simulink model "LIN_1DOF"  (R2019b)
settings: Solver=VariableStepAuto  StartTime=0.0  StopTime=600  RelTol=1e-3
InitFcn:
  | load("parameters.mat")
  | load("Coefficients.mat")
undefined symbols (not defined in the file): Dm, Dt, g, Jeq, Jp, k_pitch_, Mb, w_ramp_0N, w_ramp_0P, w_ramp_1N, w_ramp_1P
libraries: cstblocks x2
settings Model: Creator=laptop  LastModifiedBy=lbend
settings OptimizationCC: BlockReduction=off  DefaultParameterBehavior=Inlined  BufferReuse=off

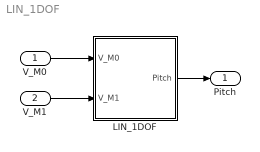
== system LIN_1DOF ==
  "V_M0 " : Inport
  V_M1 : Inport  Port=2
  LIN_1DOF : Subsystem
  Pitch : Outport
  wires:
  "V_M0 "/1 -> LIN_1DOF/1("V_M0 ")
  V_M1/1 -> LIN_1DOF/2(V_M1)
  LIN_1DOF/1(Pitch) -> Pitch/1

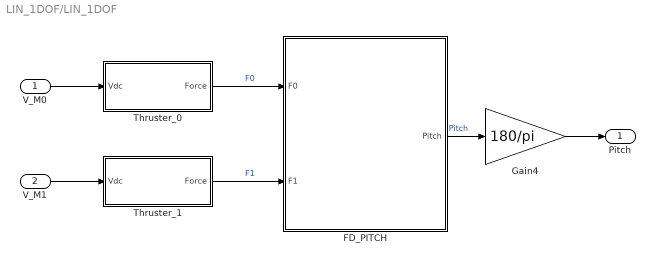
== system LIN_1DOF/LIN_1DOF ==
  "V_M0 " : Inport
  V_M1 : Inport  Port=2
  FD_PITCH : Subsystem
  Gain4 : Gain  Gain=180/pi
  Thruster_0 : Subsystem
  "Thruster_1 " : Subsystem
  Pitch : Outport
  wires:
  Thruster_0/1(Force) -> FD_PITCH/1(F0)  "F0"
  "Thruster_1 "/1(Force) -> FD_PITCH/2(F1)  "F1"
  V_M1/1 -> "Thruster_1 "/1(Vdc)
  "V_M0 "/1 -> Thruster_0/1(Vdc)
  FD_PITCH/1(Pitch) -> Gain4/1  "Pitch"
  Gain4/1 -> Pitch/1

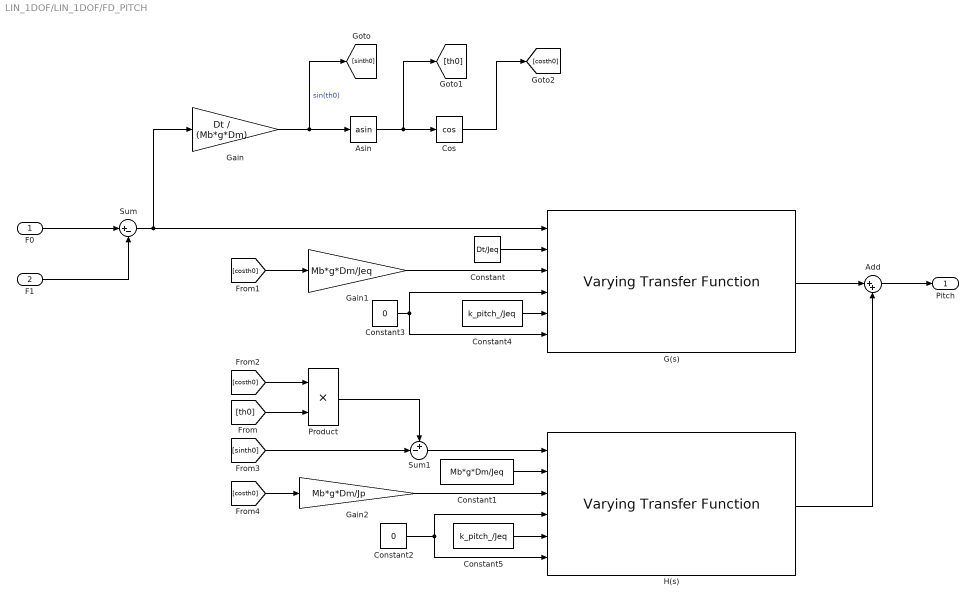
== system LIN_1DOF/LIN_1DOF/FD_PITCH ==
  F0 : Inport
  F1 : Inport  Port=2
  Add : Sum  Inputs=|++
  Asin : Trigonometry  Operator=asin
  Constant : Constant  Value=Dt/Jeq
  Constant1 : Constant  Value=Mb*g*Dm/Jeq
  Constant2 : Constant  Value=0
  Constant3 : Constant  Value=0
  Constant4 : Constant  Value=k_pitch_/Jeq
  Constant5 : Constant  Value=k_pitch_/Jeq
  Cos : Trigonometry  Operator=cos
  G(s) : cstblocks/Linear Parameter Varying/Varying Transfer Function  N=2
      settings: SourceProductName=Control System Toolbox
  Gain : Gain  Gain=Dt / (Mb*g*Dm)
  Gain1 : Gain  Gain=Mb*g*Dm/Jeq
  Gain2 : Gain  Gain=Mb*g*Dm/Jp
  H(s) : cstblocks/Linear Parameter Varying/Varying Transfer Function  N=2
      settings: SourceProductName=Control System Toolbox
  Product : Product
  Sum : Sum  Inputs=|+-
  Sum1 : Sum  Inputs=+-|
  Pitch : Outport
  wires:
  F1/1 -> Sum/2
  Constant1/1 -> H(s)/2
  Gain/1 -> [sinth0], Asin/1  "sin(th0)"
  Constant2/1 -> H(s)/6, H(s)/4
  Asin/1 -> [th0], Cos/1
  Gain2/1 -> H(s)/3
  [sinth0] -> Sum1/2
  Sum/1 -> G(s)/1, Gain/1
  Constant4/1 -> G(s)/5
  Product/1 -> Sum1/1
  [costh0] -> Gain1/1
  [th0] -> Product/2
  H(s)/1 -> Add/2
  F0/1 -> Sum/1
  [costh0] -> Product/1
  Constant/1 -> G(s)/2
  Constant3/1 -> G(s)/6, G(s)/4
  Gain1/1 -> G(s)/3
  [costh0] -> Gain2/1
  Constant5/1 -> H(s)/5
  Cos/1 -> [costh0]
  G(s)/1 -> Add/1
  Sum1/1 -> H(s)/1
  Add/1 -> Pitch/1

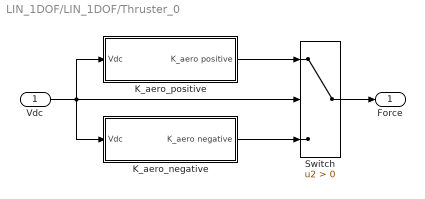
== system LIN_1DOF/LIN_1DOF/Thruster_0 ==
  Vdc : Inport
  K_aero_negative : Subsystem
  K_aero_positive : Subsystem
  Switch : Switch  Criteria=u2 > Threshold
  Force : Outport
  wires:
  Switch/1 -> Force/1
  K_aero_positive/1(K_aero positive) -> Switch/1
  Vdc/1 -> K_aero_positive/1(Vdc), K_aero_negative/1(Vdc), Switch/2
  K_aero_negative/1(K_aero negative) -> Switch/3

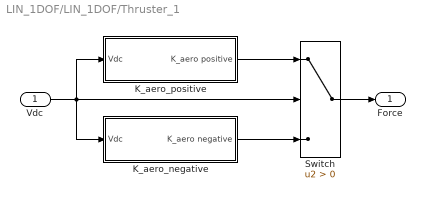
== system LIN_1DOF/LIN_1DOF/Thruster_1  ==
  Vdc : Inport
  K_aero_negative : Subsystem
  K_aero_positive : Subsystem
  Switch : Switch  Criteria=u2 > Threshold
  Force : Outport
  wires:
  Switch/1 -> Force/1
  K_aero_positive/1(K_aero positive) -> Switch/1
  Vdc/1 -> K_aero_negative/1(Vdc), Switch/2, K_aero_positive/1(Vdc)
  K_aero_negative/1(K_aero negative) -> Switch/3

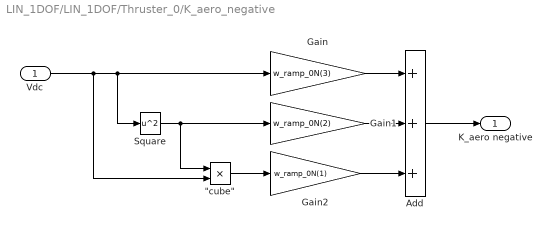
== system LIN_1DOF/LIN_1DOF/Thruster_0/K_aero_negative ==
  Vdc : Inport
  "\"cube\"" : Product  Inputs=**
  Add : Sum  Inputs=+++
  Gain : Gain  Gain=w_ramp_0N(3)
  Gain1 : Gain  Gain=w_ramp_0N(2)
  Gain2 : Gain  Gain=w_ramp_0N(1)
  Square : Math  Operator=square  SignedPower=off  SaturateOnIntegerOverflow=on
  K_aero negative : Outport
  wires:
  Vdc/1 -> "\"cube\""/2, Square/1, Gain/1
  Gain/1 -> Add/1
  Square/1 -> "\"cube\""/1, Gain1/1
  Gain1/1 -> Add/2
  Gain2/1 -> Add/3
  "\"cube\""/1 -> Gain2/1
  Add/1 -> K_aero negative/1

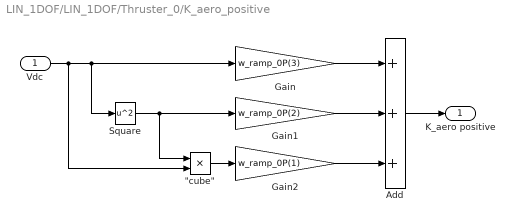
== system LIN_1DOF/LIN_1DOF/Thruster_0/K_aero_positive ==
  Vdc : Inport
  "\"cube\"" : Product  Inputs=**
  Add : Sum  Inputs=+++
  Gain : Gain  Gain=w_ramp_0P(3)
  Gain1 : Gain  Gain=w_ramp_0P(2)
  Gain2 : Gain  Gain=w_ramp_0P(1)
  Square : Math  Operator=square  SignedPower=off  SaturateOnIntegerOverflow=on
  K_aero positive : Outport
  wires:
  Vdc/1 -> Gain/1, Square/1, "\"cube\""/2
  Add/1 -> K_aero positive/1
  Gain/1 -> Add/1
  Square/1 -> "\"cube\""/1, Gain1/1
  Gain1/1 -> Add/2
  "\"cube\""/1 -> Gain2/1
  Gain2/1 -> Add/3

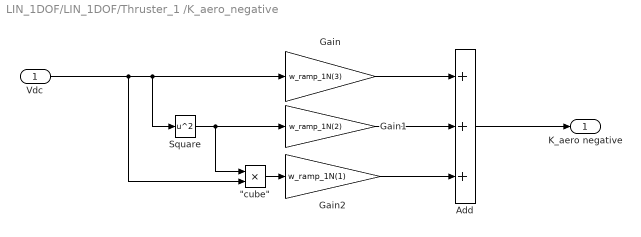
== system LIN_1DOF/LIN_1DOF/Thruster_1 /K_aero_negative ==
  Vdc : Inport
  "\"cube\"" : Product  Inputs=**
  Add : Sum  Inputs=+++
  Gain : Gain  Gain=w_ramp_1N(3)
  Gain1 : Gain  Gain=w_ramp_1N(2)
  Gain2 : Gain  Gain=w_ramp_1N(1)
  Square : Math  Operator=square  SignedPower=off  SaturateOnIntegerOverflow=on
  K_aero negative : Outport
  wires:
  Vdc/1 -> "\"cube\""/2, Square/1, Gain/1
  Gain/1 -> Add/1
  Square/1 -> "\"cube\""/1, Gain1/1
  Gain1/1 -> Add/2
  Gain2/1 -> Add/3
  "\"cube\""/1 -> Gain2/1
  Add/1 -> K_aero negative/1

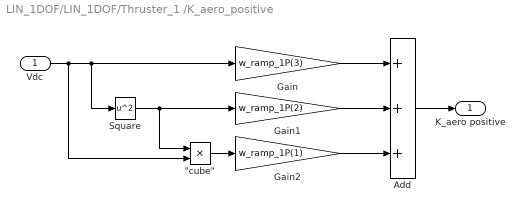
== system LIN_1DOF/LIN_1DOF/Thruster_1 /K_aero_positive ==
  Vdc : Inport
  "\"cube\"" : Product  Inputs=**
  Add : Sum  Inputs=+++
  Gain : Gain  Gain=w_ramp_1P(3)
  Gain1 : Gain  Gain=w_ramp_1P(2)
  Gain2 : Gain  Gain=w_ramp_1P(1)
  Square : Math  Operator=square  SignedPower=off  SaturateOnIntegerOverflow=on
  K_aero positive : Outport
  wires:
  Vdc/1 -> Gain/1, Square/1, "\"cube\""/2
  Add/1 -> K_aero positive/1
  Gain/1 -> Add/1
  Square/1 -> "\"cube\""/1, Gain1/1
  Gain1/1 -> Add/2
  "\"cube\""/1 -> Gain2/1
  Gain2/1 -> Add/3
